simulink model "ModelDosingUnit_FMU"  (R2020b)
settings: Solver=FixedStepAuto  StartTime=0.0  StopTime=1  FixedStep=0.010  RelTol=1e-3
settings Model: Creator=kaebi  LastModifiedBy=kaebi
settings OptimizationCC: EnhancedBackFolding=on  PassReuseOutputArgsAs=Individual arguments  ZeroExternalMemoryAtStartup=off  ZeroInternalMemoryAtStartup=off  OptimizeBlockOrder=speed  DifferentSizesBufferReuse=on  OptimizationCustomize=off  EfficientTunableParamExpr=on
settings DebuggingCC: ParameterTunabilityLossMsg=error
settings HardwareCC: ProdBitPerInt=16  ProdBitPerPointer=16  ProdBitPerSizeT=16  ProdBitPerPtrDiffT=16  ProdLargestAtomicFloat=None  ProdWordSize=8  ProdHWDeviceType=Atmel->AVR
settings SFSimCC: MATLABDynamicMemAlloc=off
settings RTWCC: Description=Run on Target Hardware  SystemTargetFile=realtime.tlc  GenCodeOnly=on  GenerateMakefile=off  TemplateMakefile=realtime.tmf  RTWVerbose=off
settings CodeAppCC: ForceParamTrailComments=on  IgnoreCustomStorageClasses=off  OperatorAnnotations=on  SimulinkDataObjDesc=on  SFDataObjDesc=on  InsertBlockDesc=on
settings STFCustomTargetCC: TargetLibSuffix=.a  MultiwordLength=256  GenerateSampleERTMain=on  ConcurrentExecutionCompliant=off  CombineOutputUpdateFcns=on  ERTCustomFileBanners=on  SupportContinuousTime=off  SupportNonInlinedSFcns=off  RemoveResetFunc=on  MATLABClassNameForMDSCustomization=Simulink.SoftwareTarget.ERTCustomization  CPPClassGenCompliant=off  GRTInterface=off  SystemTargetFile=realtime.tlc
settings ERTTargetCC: GenerateSampleERTMain=on  ParMdlRefBuildCompliant=off  CompOptLevelCompliant=off  ConcurrentExecutionCompliant=off  ModelStepFunctionPrototypeControlCompliant=off  CPPClassGenCompliant=off  UseToolchainInfoCompliant=off  ERTCustomFileTemplate=realtime_file_process.tlc

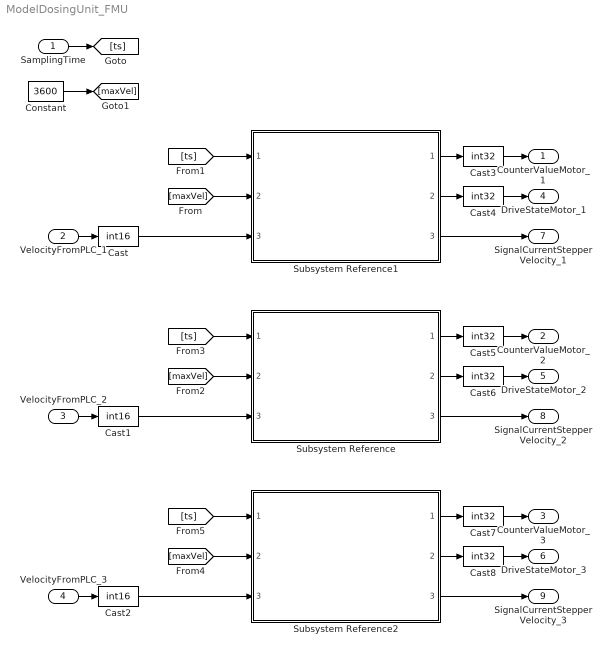
== system ModelDosingUnit_FMU ==
  SamplingTime : Inport
  VelocityFromPLC_1 : Inport  Port=2  OutDataTypeStr=int32
  VelocityFromPLC_2 : Inport  Port=3  OutDataTypeStr=int32
  VelocityFromPLC_3 : Inport  Port=4  OutDataTypeStr=int32
  Cast : DataTypeConversion  OutDataTypeStr=int16
  Cast1 : DataTypeConversion  OutDataTypeStr=int16
  Cast2 : DataTypeConversion  OutDataTypeStr=int16
  Cast{3..8} (6 alike) : DataTypeConversion  OutDataTypeStr=int32
  Constant : Constant  Value=3600
  Subsystem Reference : Subsystem  ReferencedSubsystem=SubsystemGenericDrive
  Subsystem Reference1 : Subsystem  ReferencedSubsystem=SubsystemGenericDrive
  Subsystem Reference2 : Subsystem  ReferencedSubsystem=SubsystemGenericDrive
  CounterValueMotor_1 : Outport
  CounterValueMotor_2 : Outport  Port=2
  CounterValueMotor_3 : Outport  Port=3
  DriveStateMotor_1 : Outport  Port=4
  DriveStateMotor_2 : Outport  Port=5
  DriveStateMotor_3 : Outport  Port=6
  SignalCurrentStepperVelocity_1 : Outport  Port=7
  SignalCurrentStepperVelocity_2 : Outport  Port=8
  SignalCurrentStepperVelocity_3 : Outport  Port=9
  wires:
  SamplingTime/1 -> [ts]
  Constant/1 -> [maxVel]
  [ts] -> Subsystem Reference1/1
  VelocityFromPLC_1/1 -> Cast/1
  [maxVel] -> Subsystem Reference1/2
  Subsystem Reference1/1 -> Cast3/1
  Subsystem Reference1/2 -> Cast4/1
  Subsystem Reference1/3 -> SignalCurrentStepperVelocity_1/1
  Subsystem Reference/3 -> SignalCurrentStepperVelocity_2/1
  Subsystem Reference/2 -> Cast6/1
  Subsystem Reference/1 -> Cast5/1
  [maxVel] -> Subsystem Reference/2
  VelocityFromPLC_2/1 -> Cast1/1
  [ts] -> Subsystem Reference/1
  [ts] -> Subsystem Reference2/1
  VelocityFromPLC_3/1 -> Cast2/1
  [maxVel] -> Subsystem Reference2/2
  Subsystem Reference2/1 -> Cast7/1
  Subsystem Reference2/2 -> Cast8/1
  Subsystem Reference2/3 -> SignalCurrentStepperVelocity_3/1
  Cast/1 -> Subsystem Reference1/3
  Cast1/1 -> Subsystem Reference/3
  Cast2/1 -> Subsystem Reference2/3
  Cast3/1 -> CounterValueMotor_1/1
  Cast4/1 -> DriveStateMotor_1/1
  Cast5/1 -> CounterValueMotor_2/1
  Cast6/1 -> DriveStateMotor_2/1
  Cast7/1 -> CounterValueMotor_3/1
  Cast8/1 -> DriveStateMotor_3/1
